simulink model "sig_mod_block_5"  (R2019a)
settings: Solver=VariableStepAuto  StartTime=0.0  StopTime=10.0  RelTol=1e-3
undefined symbols (not defined in the file): intmax, mod_fcn, sig_in, sig_mod_enabled, sig_out
libraries: simulink x3
settings Model: Creator=a3bawa  LastModifiedBy=a3bawa

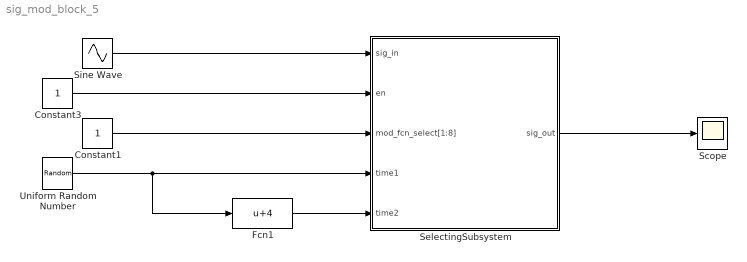
== system sig_mod_block_5 ==
  Constant1 : Constant
  Constant3 : Constant
  Fcn1 : Fcn  Expr=u+4
  Scope : Scope
  SelectingSubsystem : Subsystem
  Sine Wave : Sin  SampleTime=0
  Uniform Random Number : UniformRandomNumber  Minimum=0  Maximum=6  Seed=randi(intmax)  SampleTime=0.1
  wires:
  Uniform Random Number/1 -> Fcn1/1, SelectingSubsystem/4(time1)
  Sine Wave/1 -> SelectingSubsystem/1(sig_in)
  Constant3/1 -> SelectingSubsystem/2(en)
  Constant1/1 -> SelectingSubsystem/3(mod_fcn_select[1:8])
  Fcn1/1 -> SelectingSubsystem/5(time2)
  SelectingSubsystem/1(sig_out) -> Scope/1

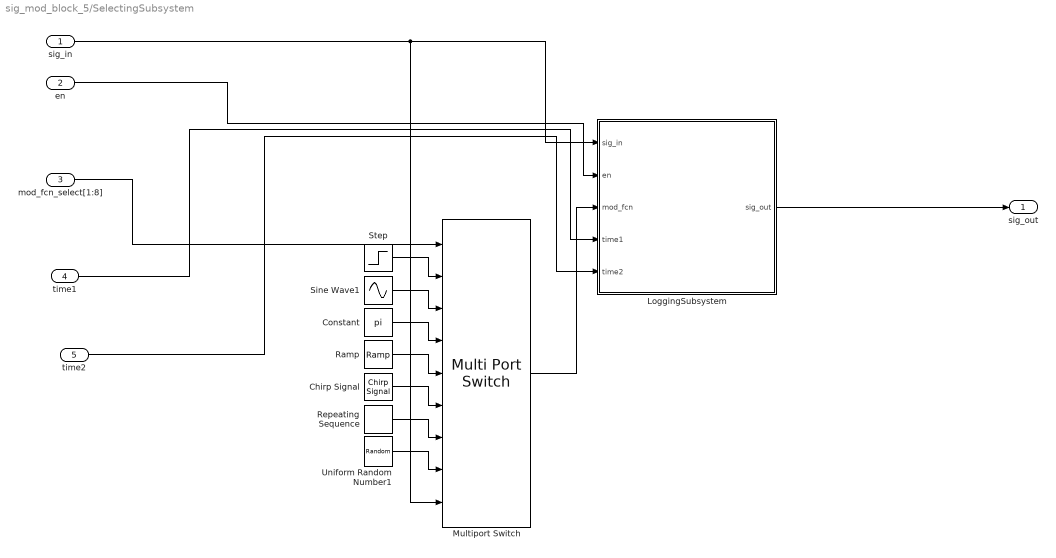
== system sig_mod_block_5/SelectingSubsystem ==
  sig_in : Inport
  en : Inport  Port=2
  mod_fcn_select[1:8] : Inport  Port=3
  time1 : Inport  Port=4
  time2 : Inport  Port=5
  Chirp Signal : simulink/Sources/Chirp Signal  f1=1  T=10  f2=1000
  Constant : Constant  Value=pi
  LoggingSubsystem : Subsystem
  Multiport Switch : MultiPortSwitch  Inputs=7  DataPortForDefault=Additional data port  DiagnosticForDefault=Warning
  Ramp : simulink/Sources/Ramp  slope=1  start=5  InitialOutput=0
  Repeating Sequence : simulink/Sources/Repeating Sequence  rep_seq_t=[0 2]  rep_seq_y=[0 1]
  Sine Wave1 : Sin  Frequency=1000  SampleTime=0
  Step : Step  Time=5  SampleTime=0
  Uniform Random Number1 : UniformRandomNumber  Minimum=-10  Maximum=10  Seed=randi(intmax)  SampleTime=0.1
  sig_out : Outport
  wires:
  Constant/1 -> Multiport Switch/4
  Chirp Signal/1 -> Multiport Switch/6
  Ramp/1 -> Multiport Switch/5
  sig_in/1 -> LoggingSubsystem/1(sig_in), Multiport Switch/9
  Sine Wave1/1 -> Multiport Switch/3
  Repeating Sequence/1 -> Multiport Switch/7
  mod_fcn_select[1:8]/1 -> Multiport Switch/1
  Multiport Switch/1 -> LoggingSubsystem/3(mod_fcn)
  Uniform Random Number1/1 -> Multiport Switch/8
  en/1 -> LoggingSubsystem/2(en)
  Step/1 -> Multiport Switch/2
  LoggingSubsystem/1(sig_out) -> sig_out/1
  time1/1 -> LoggingSubsystem/4(time1)
  time2/1 -> LoggingSubsystem/5(time2)

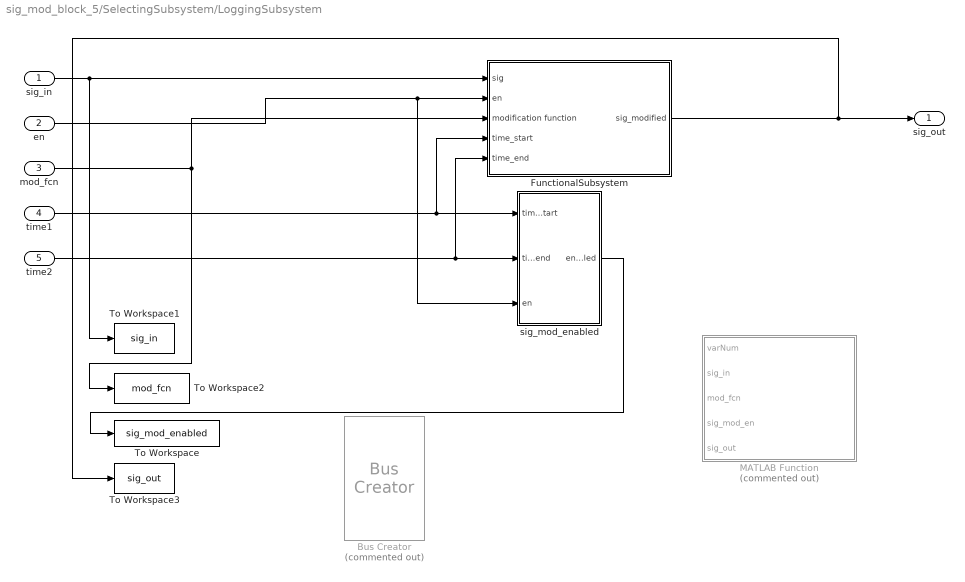
== system sig_mod_block_5/SelectingSubsystem/LoggingSubsystem ==
  sig_in : Inport
  en : Inport  Port=2
  mod_fcn : Inport  Port=3
  time1 : Inport  Port=4
  time2 : Inport  Port=5
  Bus Creator : BusCreator  Commented=on  Inputs=sig_in,mod_fcn,sig_mod_enabled,sig_out
  FunctionalSubsystem : Subsystem  TreatAsAtomicUnit=on
  MATLAB Function : MATLAB Function  Commented=on  TreatAsAtomicUnit=on
  To Workspace : ToWorkspace  VariableName=sig_mod_enabled  SaveFormat=Timeseries  SampleTime=-1
  To Workspace1 : ToWorkspace  VariableName=sig_in  SaveFormat=Timeseries  SampleTime=-1
  To Workspace2 : ToWorkspace  VariableName=mod_fcn  SaveFormat=Timeseries  SampleTime=-1
  To Workspace3 : ToWorkspace  VariableName=sig_out  SaveFormat=Timeseries  SampleTime=-1
  sig_mod_enabled : Subsystem
  sig_out : Outport
  wires:
  FunctionalSubsystem/1(sig_modified) -> sig_out/1, To Workspace3/1
  sig_in/1 -> FunctionalSubsystem/1(sig), To Workspace1/1
  en/1 -> FunctionalSubsystem/2(en), sig_mod_enabled/3(en)
  sig_mod_enabled/1(enabled) -> To Workspace/1
  mod_fcn/1 -> FunctionalSubsystem/3(modification function), To Workspace2/1
  time1/1 -> sig_mod_enabled/1(time_start), FunctionalSubsystem/4(time_start)
  time2/1 -> FunctionalSubsystem/5(time_end), sig_mod_enabled/2(time_end)

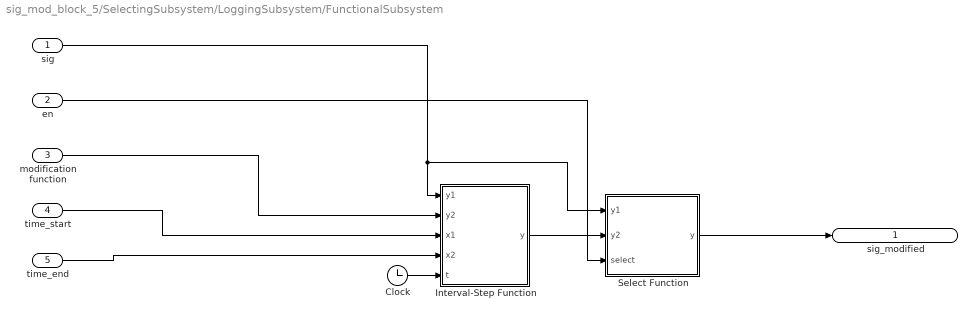
== system sig_mod_block_5/SelectingSubsystem/LoggingSubsystem/FunctionalSubsystem ==
  sig : Inport
  en : Inport  Port=2
  modification function : Inport  Port=3
  time_start : Inport  Port=4
  time_end : Inport  Port=5
  Clock : Clock
  Interval-Step Function : MATLAB Function  TreatAsAtomicUnit=on
  Select Function : MATLAB Function  TreatAsAtomicUnit=on
  sig_modified : Outport
  wires:
  Interval-Step Function/1(y) -> Select Function/2(y2)
  Clock/1 -> Interval-Step Function/5(t)
  en/1 -> Select Function/3(select)
  sig/1 -> Interval-Step Function/1(y1), Select Function/1(y1)
  Select Function/1(y) -> sig_modified/1
  modification function/1 -> Interval-Step Function/2(y2)
  time_start/1 -> Interval-Step Function/3(x1)
  time_end/1 -> Interval-Step Function/4(x2)

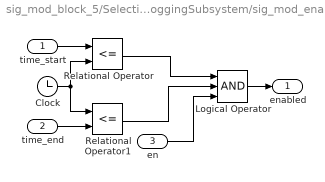
== system sig_mod_block_5/SelectingSubsystem/LoggingSubsystem/sig_mod_enabled ==
  time_start : Inport
  time_end : Inport  Port=2
  en : Inport  Port=3
  Clock : Clock
  Logical Operator : Logic  Inputs=3  AllPortsSameDT=off  OutDataTypeStr=boolean
  Relational Operator : RelationalOperator  Operator=<=  OutDataTypeStr=boolean  RndMeth=Simplest
  Relational Operator1 : RelationalOperator  Operator=<=  OutDataTypeStr=boolean  RndMeth=Simplest
  enabled : Outport
  wires:
  Relational Operator1/1 -> Logical Operator/2
  Clock/1 -> Relational Operator1/1, Relational Operator/2
  time_end/1 -> Relational Operator1/2
  Relational Operator/1 -> Logical Operator/1
  time_start/1 -> Relational Operator/1
  Logical Operator/1 -> enabled/1
  en/1 -> Logical Operator/3

== matlab function sig_mod_block_5/SelectingSubsystem/LoggingSubsystem/FunctionalSubsystem/Interval-Step Function ==
  data: y1 input; y output; y2 input; x1 input; x2 input; t input
function y = fcn(y1,y2,x1,x2,t)

if (x1<=t)&&(t<x2)
    y=y2;
else
    y=y1;
end

== matlab function sig_mod_block_5/SelectingSubsystem/LoggingSubsystem/MATLAB Function ==
  data: varNum input; sig_in input; mod_fcn input; sig_mod_en input; sig_out input
function saveToVar(varNum,sig_in,mod_fcn,sig_mod_en,sig_out)

== matlab function sig_mod_block_5/SelectingSubsystem/LoggingSubsystem/FunctionalSubsystem/Select Function ==
  data: y1 input; y output; y2 input; select input
function y = fcn(y1,y2,select)

if select>=1
    y=y2;
else
    y=y1;
end
